simulink model "chap02_03_46_mdl"  (R2013b)
settings: Solver=ode45  StartTime=0.0  StopTime=10.0  RelTol=1e-3
settings Model: Creator=Administrator  LastModifiedBy=sunzx.fnst

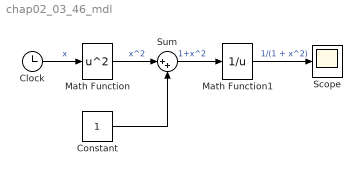
== system chap02_03_46_mdl ==
  Clock : Clock
  Constant : Constant
  Math Function : Math  Operator=square  OutputSignalType=real  SaturateOnIntegerOverflow=on
  Math Function1 : Math  Operator=reciprocal  OutputSignalType=real  SaturateOnIntegerOverflow=on
  Scope : Scope
      settings: ShowLegends=on
  Sum : Sum  Inputs=|++
  wires:
  Clock/1 -> Math Function/1  "x"
  Math Function/1 -> Sum/1  "x^2"
  Constant/1 -> Sum/2
  Sum/1 -> Math Function1/1  "1+x^2"
  Math Function1/1 -> Scope/1  "1/(1 + x^2)"
